simulink model "Projekt"  (R2016a)
settings: Solver=VariableStepAuto  StartTime=0.0  StopTime=2  MaxStep=0.01  RelTol=1e-4
values from neighbouring files (symbols this model uses):
  b = 0.000931    [Model.m]    (also in Projekt_disturbance.m; Rlocus.m = 3.5077e-06)
  J = 0.3    [Model.m]    (also in Projekt_disturbance.m = 0.00567; Rlocus.m = 3.2284e-06)
  Kb = 0.509    [Model.m]    (also in Projekt_disturbance.m)
  Km = 0.509    [Model.m]    (also in Projekt_disturbance.m)
  La = 0.0034    [Model.m]    (also in Projekt_disturbance.m)
  Ra = 7.101    [Model.m]    (also in Projekt_disturbance.m)
undefined symbols (not defined in the file or in its folder): Scaling
libraries: simulink x1
settings Model: Creator=Kristian  LastModifiedBy=Kristian
settings DataIOCC: LimitDataPoints=on  SaveOutput=off  SaveTime=off
settings OptimizationCC: ExpressionDepthLimit=2147483647  LifeSpan=1
settings DebuggingCC: UnderspecifiedInitializationDetection=Classic  MergeDetectMultiDrivingBlocksExec=none  FcnCallInpInsideContextMsg=EnableAllAsWarning  AllowSymbolicDim=off  StateNameClashWarn=warning
settings GRTTargetCC: CombineOutputUpdateFcns=off  GRTInterface=on

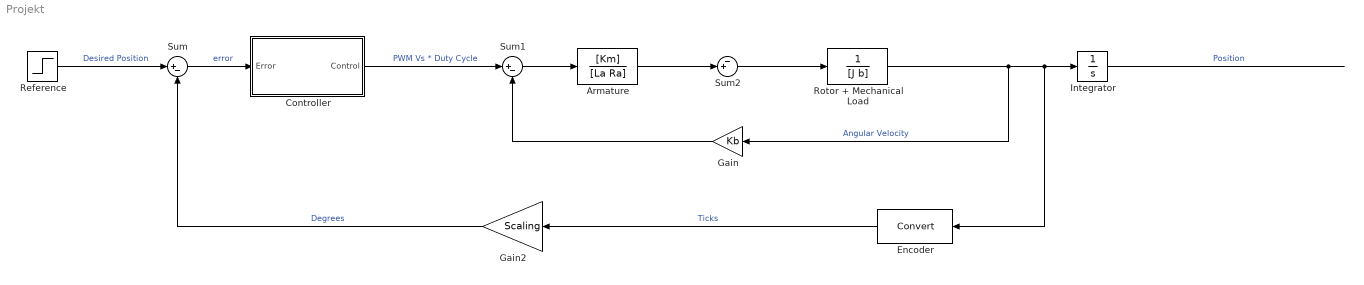
== system Projekt ==
  Armature : TransferFcn  Numerator=[Km]  Denominator=[La Ra]
  Controller : Subsystem
  "Encoder\t" : DataTypeConversion
  Gain : Gain  Gain=Kb
  Gain2 : Gain  Gain=Scaling
  Integrator : Integrator
  Reference : Step  SampleTime=0
  Rotor + Mechanical Load : TransferFcn  Denominator=[J b]
  Sum : Sum  Inputs=|+-
  Sum1 : Sum  Inputs=|+-
  Sum2 : Sum  Inputs=-+|
  wires:
  Reference/1 -> Sum/1  "Desired Position"
  Integrator/1 -> ?  "Position"
  Sum/1 -> Controller/1(Error)  "error"
  Controller/1(Control) -> Sum1/1  "PWM Vs * Duty Cycle"
  Armature/1 -> Sum2/2
  Sum2/1 -> Rotor + Mechanical Load/1
  ? -> Sum2/1  "Disturbance Torque"
  Sum1/1 -> Armature/1
  Gain/1 -> Sum1/2
  Rotor + Mechanical Load/1 -> "Encoder\t"/1, Integrator/1, Gain/1  "Angular Velocity"
  Gain2/1 -> Sum/2  "Degrees"
  "Encoder\t"/1 -> Gain2/1  "Ticks"

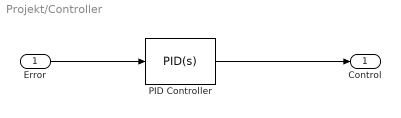
== system Projekt/Controller ==
  Error : Inport
  PID Controller : simulink/Continuous/PID Controller  Controller=PID  TimeDomain=Continuous-time  SampleTime=-1  IntegratorMethod=Forward Euler  FilterMethod=Forward Euler  Form=Parallel  UseFilter=on  ControllerParametersSource=internal  P=1.2  I=22  D=0.02  N=20  InitialConditionSource=internal  InitialConditionForIntegrator=0  InitialConditionForFilter=0  ExternalReset=none  LimitOutput=off  UpperSaturationLimit=inf  LowerSaturationLimit=-inf  LinearizeAsGain=on  AntiWindupMode=none  Kb=1  TrackingMode=off  Kt=1  PParamMin=[]  PParamMax=[]  IParamMin=[]  IParamMax=[]  DParamMin=[]  DParamMax=[]  NParamMin=[]  NParamMax=[]  KbParamMin=[]  KbParamMax=[]  KtParamMin=[]  KtParamMax=[]  POutMin=[]  POutMax=[]  IOutMin=[]  IOutMax=[]  DOutMin=[]  DOutMax=[]  NOutMin=[]  NOutMax=[]  KbOutMin=[]  KbOutMax=[]  KtOutMin=[]  KtOutMax=[]  IntegratorOutMin=[]  IntegratorOutMax=[]  FilterOutMin=[]  FilterOutMax=[]  SumOutMin=[]  SumOutMax=[]  SumI1OutMin=[]  SumI1OutMax=[]  SumI2OutMin=[]  SumI2OutMax=[]  SumI3OutMin=[]  SumI3OutMax=[]  SumDOutMin=[]  SumDOutMax=[]  SaturationOutMin=[]  SaturationOutMax=[]  IntegratorContinuousStateAttributes=''  IntegratorStateMustResolveToSignalObject=off  IntegratorRTWStateStorageClass=Auto  FilterContinuousStateAttributes=''  FilterStateMustResolveToSignalObject=off  FilterRTWStateStorageClass=Auto  DifferentiatorICPrevScaledInput=0  DifferentiatorOutMin=[]  DifferentiatorOutMax=[]
  Control : Outport
  wires:
  Error/1 -> PID Controller/1
  PID Controller/1 -> Control/1
